simulink model "slett"  (Simulink 7.9)
settings: Solver=ode45  StartTime=0.0  StopTime=10.0  RelTol=1e-3
settings Model: Creator=simena  LastModifiedBy=simena

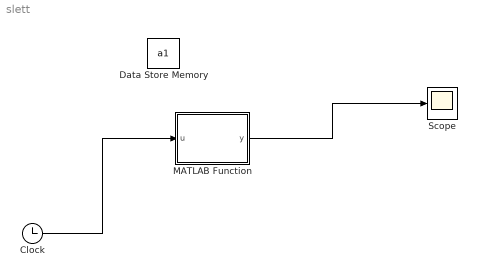
== system slett ==
  Clock : Clock
  Data Store Memory : DataStoreMemory  DataStoreName=a1  ReadBeforeWriteMsg=warning  WriteAfterWriteMsg=warning  WriteAfterReadMsg=warning  OutDataTypeStr=double
  MATLAB Function : MATLAB Function  TreatAsAtomicUnit=on
  Scope : Scope
  wires:
  Clock/1 -> MATLAB Function/1(u)
  MATLAB Function/1(y) -> Scope/1

== matlab function MATLAB Function ==
  data: u input double; y output double; a1 data_store_memory double
function y = fcn(u)
%#codegen
global a1;

a1=a1+u;
y = a1;
